simulink model "deney3-1"  (R2023b)
settings: Solver=VariableStepAuto  StartTime=0.0  StopTime=10.0  RelTol=1e-3
libraries: dspfdesign x1, commrandsrc3 x1
settings Model: Creator=FEYZA  LastModifiedBy=msi

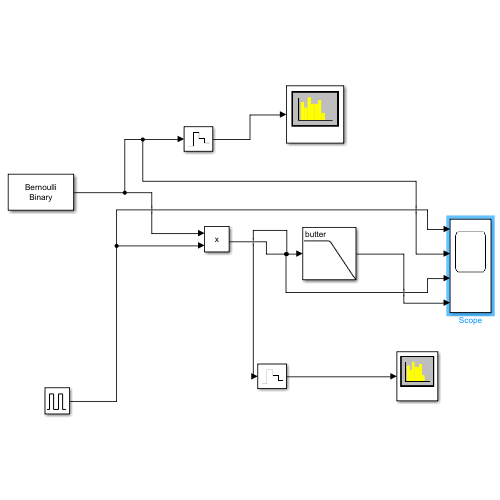
[thumbnail: Simulink's stored preview of the top-level diagram]
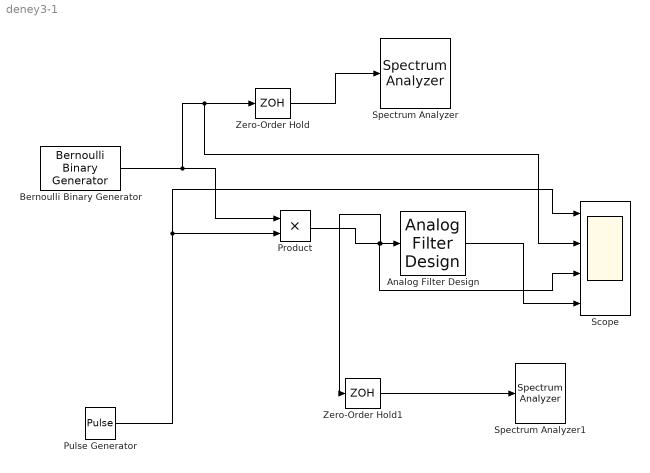
== system deney3-1 ==
  Analog Filter Design : dspfdesign/Analog Filter Design  method=Butterworth  filttype=Lowpass  N=8  Wlo=30  Whi=80  Rp=2  Rs=40
  Bernoulli Binary Generator : commrandsrc3/Bernoulli Binary Generator  ProbabilityOfZero=0.5  SeedSource=Auto  Seed=0  SampleTime=1/1000  SamplesPerFrame=1  OutputDataType=double  SimulateUsing=Code generation
  Product : Product
  Pulse Generator : DiscretePulseGenerator  PulseType=Time based  Amplitude=5  Period=1/1000  PulseWidth=50
  Scope : Scope  NumInputPorts=4
  Spectrum Analyzer : SpectrumAnalyzer  WindowPosition=[1.000000,49.000000,1536.000000,793.000000,]  Visible=on  ScopeFrameLocation=window  Method=Welch  Span=1000  StartFrequency=-500  StopFrequency=500  YLimits=[-16.54787588,28.48685306]
  Spectrum Analyzer1 : SpectrumAnalyzer  WindowPosition=[1.000000,49.000000,1536.000000,793.000000,]  Visible=on  ScopeFrameLocation=window  Method=Welch  Span=1000  StartFrequency=-500  StopFrequency=500  YLimits=[-2.56847579,42.46625315]  ShowLegend=on  SelectedToolstripTab=spectrumAnalyzerToolstrip.measurementsTab
  Zero-Order Hold : ZeroOrderHold  SampleTime=-1
  Zero-Order Hold1 : ZeroOrderHold  SampleTime=-1
  wires:
  Bernoulli Binary Generator/1 -> Scope/2, Zero-Order Hold/1, Product/1
  Pulse Generator/1 -> Scope/1, Product/2
  Analog Filter Design/1 -> Scope/4
  Product/1 -> Scope/3, Zero-Order Hold1/1, Analog Filter Design/1
  Zero-Order Hold1/1 -> Spectrum Analyzer1/1
  Zero-Order Hold/1 -> Spectrum Analyzer/1
